simulink model "ESTteam33"  (R2024b)
settings: Solver=FixedStepAuto  StartTime=0.0  StopTime=stopt  FixedStep=deltat  MaxStep=0.05  RelTol=1e-3
InitFcn:
  | clear all;
  | close all;
  | clc;
  | 
  | % add the data and script directories
  | addpath('data','scripts');
  | 
  | % load the constants (units)
  | constants;
  | 
  | % load the simulation parameters
  | preprocessing;
StopFcn:
  | postprocessing;
values from neighbouring files (symbols this model uses):
  aExtraction = eta_extr    (= 0.8439)    [preprocessing.m]
  bStorage = 0    [preprocessing.m]
  deltat = 5*unit("min")    [preprocessing.m]
  EStorageInitial = EStorageMax/2    (= 1000000000)    [preprocessing.m]
  EStorageMax = 2*10e8    (= 2000000000)    [preprocessing.m]
  EStorageMin = EStorageMax/20    (= 100000000)    [preprocessing.m]
  eta_converter = 0.97    [preprocessing.m]
  L = 0.11 * 29    (= 3.19)    [preprocessing.m]
  L_demand = 10    [preprocessing.m]
  N_sphere = 9    [preprocessing.m]
  r_sph = 10    [preprocessing.m]
  Rprime = 0.1181    [preprocessing.m]
  V = 320e3    (= 320000)    [preprocessing.m]
settings Model: Creator=joche  LastModifiedBy=yujingze
settings DataIOCC: SaveFormat=Array  SaveOutput=off  ReturnWorkspaceOutputs=off
settings OptimizationCC: ReuseModelBlockBuffer=off
settings ModelReferenceCC: EnableRefExpFcnMdlSchedulingChecks=on
settings RTWCC: GPUComputeCapability=3.5

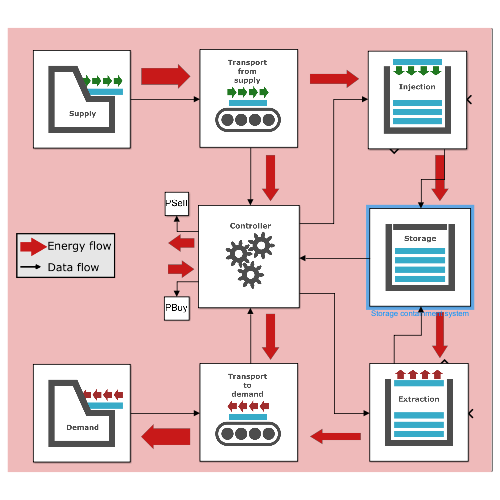
[thumbnail: Simulink's stored preview of the top-level diagram]
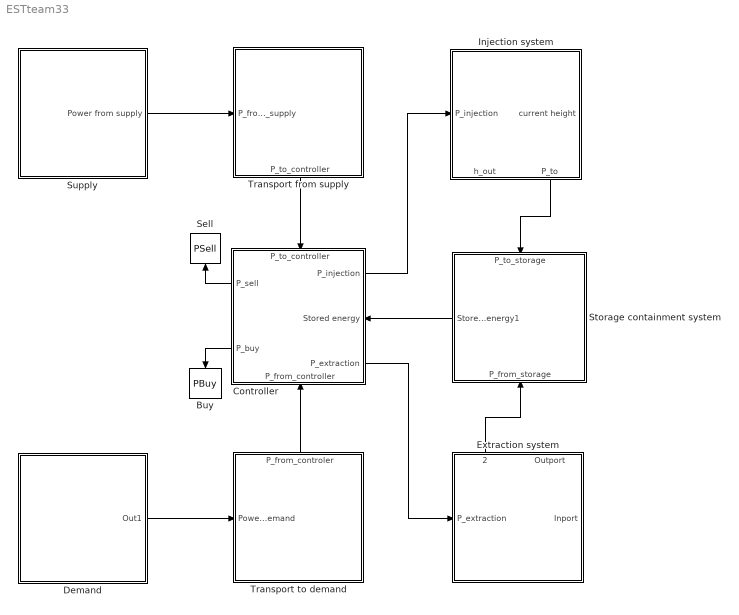
== system ESTteam33 ==
  Buy : ToWorkspace  VariableName=PBuy  SampleTime=-1
  Controller : Subsystem
      settings: PortSchema="{\"entries\":[{\"content\":{\"sides\":[{\"content\":{\"connectorIds\":[\"Out3\",\"Out4\"]},\"type\":\"ConnectorPlacement.EquallySpacedRectSide\",\"uuid\":\"4daf33ce-c96a-4783-b5c4-228eed953e01\"},{\"content\":{\"connectorIds\":[\"Out1\",\"In3\",\"Out2\"],\"side\":\"RIGHT\"},\"type\":\"ConnectorPlacement.EquallySpacedRectSide\",\"uuid\":\"e9942e50-8467-4af8-b79b-80636cbc76e5\"},{\"content\":{\"connectorIds\":[\"In1\"],\"side\":\"TOP\"},\"type\":\"ConnectorPlacement.EquallySpacedRectSide\",\"uuid\":\"f315e931-d69b-4751-b712-f89c6c81baeb\"},{\"content\":{\"connectorIds\":[\"In2\"],\"side\":\"BOTTOM\"},\"type\":\"ConnectorPlacement.EquallySpacedRectSide\",\"uuid\":\"44715ee6-5cd5-4669-bcb9-5ed7c869bdb3\"}]},\"type\":\"ConnectorPlacement.EquallySpacedConnector\",\"uuid\":\"fff48899-944b-4064-b7d7-ecc12144fb48\"}],\"packageUris\":[\"http://schema.mathworks.com/mf0/Connector/R2020b\"],\"version\":\"1.0\"}"
      mask Display: image('$imagefile'); % Use "Edit Image" on toolstrip to change.
  Demand : Subsystem
      mask Display: image('$imagefile'); % Use "Edit Image" on toolstrip to change.
  Extraction system : Subsystem
      settings: PortSchema="{\"entries\":[{\"content\":{\"sides\":[{\"content\":{\"connectorIds\":[\"In1\"]},\"type\":\"ConnectorPlacement.EquallySpacedRectSide\",\"uuid\":\"05c5933d-55fc-4e06-853f-fc26d42905f9\"},{\"content\":{\"connectorIds\":[\"In2\"],\"side\":\"RIGHT\"},\"type\":\"ConnectorPlacement.EquallySpacedRectSide\",\"uuid\":\"327426c5-31d5-498b-a2bd-83e49353408c\"},{\"content\":{\"side\":\"TOP\"},\"type\":\"ConnectorPlacement.EquallySpacedRectSide\",\"uuid\":\"55306cf3-a3de-4385-a5ae-b8600ecdd5a2\"},{\"content\":{\"connectorIds\":[\"Out1\",\"Out2\"],\"side\":\"BOTTOM\"},\"type\":\"ConnectorPlacement.EquallySpacedRectSide\",\"uuid\":\"08fcc9c3-40d3-4ac6-b914-dfeef6039ffb\"}]},\"type\":\"ConnectorPlacement.EquallySpacedConnector\",\"uuid\":\"cb35d5ba-e8c6-462c-b7b2-fe8356d4b0a1\"}],\"packageUris\":[\"http://schema.mathworks.com/mf0/Connector/R2020b\"],\"version\":\"1.0\"}"
      mask Display: image('$imagefile'); % Use "Edit Image" on toolstrip to change.
  Injection system : Subsystem
      settings: PortSchema="{\"entries\":[{\"content\":{\"sides\":[{\"content\":{\"connectorIds\":[\"In1\"]},\"type\":\"ConnectorPlacement.EquallySpacedRectSide\",\"uuid\":\"05c5933d-55fc-4e06-853f-fc26d42905f9\"},{\"content\":{\"connectorIds\":[\"In2\"],\"side\":\"RIGHT\"},\"type\":\"ConnectorPlacement.EquallySpacedRectSide\",\"uuid\":\"327426c5-31d5-498b-a2bd-83e49353408c\"},{\"content\":{\"connectorIds\":[\"Out1\",\"Out2\"],\"side\":\"TOP\"},\"type\":\"ConnectorPlacement.EquallySpacedRectSide\",\"uuid\":\"55306cf3-a3de-4385-a5ae-b8600ecdd5a2\"},{\"content\":{\"side\":\"BOTTOM\"},\"type\":\"ConnectorPlacement.EquallySpacedRectSide\",\"uuid\":\"08fcc9c3-40d3-4ac6-b914-dfeef6039ffb\"}]},\"type\":\"ConnectorPlacement.EquallySpacedConnector\",\"uuid\":\"cb35d5ba-e8c6-462c-b7b2-fe8356d4b0a1\"}],\"packageUris\":[\"http://schema.mathworks.com/mf0/Connector/R2020b\"],\"version\":\"1.0\"}"
      mask Display: image('$imagefile'); % Use "Edit Image" on toolstrip to change.
  Sell : ToWorkspace  VariableName=PSell  SampleTime=-1
  Storage containment system : Subsystem
      settings: PortSchema="{\"entries\":[{\"content\":{\"sides\":[{\"content\":{\"connectorIds\":[\"Out1\"]},\"type\":\"ConnectorPlacement.EquallySpacedRectSide\",\"uuid\":\"0ba48424-33b9-4934-970f-64fe5d8b070e\"},{\"content\":{\"side\":\"RIGHT\"},\"type\":\"ConnectorPlacement.EquallySpacedRectSide\",\"uuid\":\"9cde340f-8f39-4499-9a12-5e1623737660\"},{\"content\":{\"connectorIds\":[\"In1\"],\"side\":\"TOP\"},\"type\":\"ConnectorPlacement.EquallySpacedRectSide\",\"uuid\":\"2af8db04-7fd0-4902-8637-8dc00edb4598\"},{\"content\":{\"connectorIds\":[\"In2\"],\"side\":\"BOTTOM\"},\"type\":\"ConnectorPlacement.EquallySpacedRectSide\",\"uuid\":\"e21ea806-d777-41a3-a53f-556fae66854b\"}]},\"type\":\"ConnectorPlacement.EquallySpacedConnector\",\"uuid\":\"4e2ddb36-4db3-4ab4-858b-ebb8ccefeb1f\"}],\"packageUris\":[\"http://schema.mathworks.com/mf0/Connector/R2020b\"],\"version\":\"1.0\"}"
      mask Display: image('$imagefile'); % Use "Edit Image" on toolstrip to change.
  Supply : Subsystem
      mask Display: image('$imagefile'); % Use "Edit Image" on toolstrip to change.
  Transport from supply : Subsystem
      settings: PortSchema="{\"entries\":[{\"content\":{\"sides\":[{\"content\":{\"connectorIds\":[\"In1\"]},\"type\":\"ConnectorPlacement.EquallySpacedRectSide\",\"uuid\":\"31329006-3d36-4d93-9c44-7503a515d397\"},{\"content\":{\"connectorIds\":[],\"side\":\"RIGHT\"},\"type\":\"ConnectorPlacement.EquallySpacedRectSide\",\"uuid\":\"aba139c7-f9b6-4881-a56b-a4cbbedacd88\"},{\"content\":{\"connectorIds\":[],\"side\":\"TOP\"},\"type\":\"ConnectorPlacement.EquallySpacedRectSide\",\"uuid\":\"e683eb73-7a35-4160-9c39-da83856a6278\"},{\"content\":{\"connectorIds\":[\"Out1\"],\"side\":\"BOTTOM\"},\"type\":\"ConnectorPlacement.EquallySpacedRectSide\",\"uuid\":\"1170dd18-447c-437f-9043-6812c2877331\"}]},\"type\":\"ConnectorPlacement.EquallySpacedConnector\",\"uuid\":\"804af608-1d70-444f-af69-e05f19bf98f3\"}],\"packageUris\":[\"http://schema.mathworks.com/mf0/Connector/R2020b\"],\"version\":\"1.0\"}"
      mask Display: image('$imagefile'); % Use "Edit Image" on toolstrip to change.
  Transport to demand : Subsystem
      settings: PortSchema="{\"entries\":[{\"content\":{\"sides\":[{\"content\":{\"connectorIds\":[\"In1\"]},\"type\":\"ConnectorPlacement.EquallySpacedRectSide\",\"uuid\":\"31329006-3d36-4d93-9c44-7503a515d397\"},{\"content\":{\"connectorIds\":[],\"side\":\"RIGHT\"},\"type\":\"ConnectorPlacement.EquallySpacedRectSide\",\"uuid\":\"aba139c7-f9b6-4881-a56b-a4cbbedacd88\"},{\"content\":{\"connectorIds\":[\"Out1\"],\"side\":\"TOP\"},\"type\":\"ConnectorPlacement.EquallySpacedRectSide\",\"uuid\":\"e683eb73-7a35-4160-9c39-da83856a6278\"},{\"content\":{\"connectorIds\":[],\"side\":\"BOTTOM\"},\"type\":\"ConnectorPlacement.EquallySpacedRectSide\",\"uuid\":\"c378138f-7233-4483-870c-40a69b3495ee\"}]},\"type\":\"ConnectorPlacement.EquallySpacedConnector\",\"uuid\":\"804af608-1d70-444f-af69-e05f19bf98f3\"}],\"packageUris\":[\"http://schema.mathworks.com/mf0/Connector/R2020b\"],\"version\":\"1.0\"}"
      mask Display: image('$imagefile'); % Use "Edit Image" on toolstrip to change.
  wires:
  Supply/1(Power from supply) -> Transport from supply/1(P_from_supply)
  Transport from supply/1(P_to_controller) -> Controller/1(P_to_controller)
  Transport to demand/1(P_from_controler) -> Controller/2(P_from_controller)
  Demand/1(Out1) -> Transport to demand/1(Power to demand)
  Controller/3(P_sell) -> Sell/1
  Controller/2(P_extraction) -> Extraction system/2(P_extraction)
  Injection system/1(P_to) -> Storage containment system/1(P_to_storage)
  Extraction system/2(P_from_storage) -> Storage containment system/2(P_from_storage)
  Storage containment system/1(Stored energy1) -> Controller/3(Stored energy)
  Controller/1(P_injection) -> Injection system/2(P_injection)
  Controller/4(P_buy) -> Buy/1

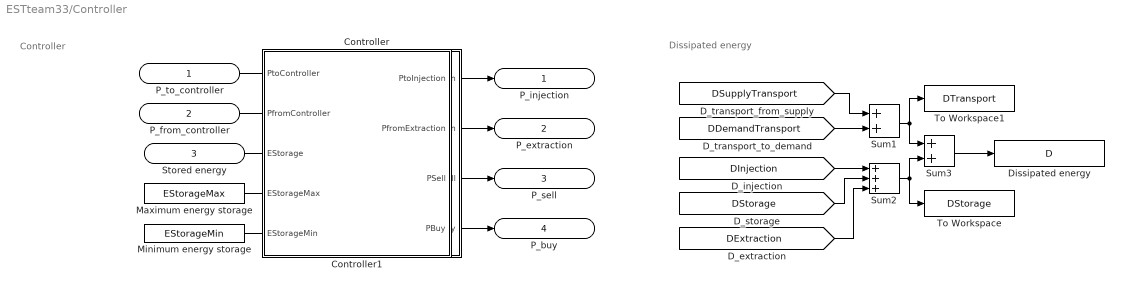
== system ESTteam33/Controller ==
  note: Dissipated energy
  note: Controller
  P_to_controller : Inport
  P_from_controller : Inport  Port=2
  Stored energy : Inport  Port=3
  Controller : MATLAB Function  TreatAsAtomicUnit=on
  Controller1 : MATLAB Function  TreatAsAtomicUnit=on
  Dissipated energy : ToWorkspace  VariableName=D  SampleTime=-1
  Maximum energy storage : Constant  Value=EStorageMax
  Minimum energy storage : Constant  Value=EStorageMin
  Sum1 : Sum
  Sum2 : Sum  Inputs=+++
  Sum3 : Sum
  To Workspace : ToWorkspace  VariableName=DStorage  SampleTime=-1
  To Workspace1 : ToWorkspace  VariableName=DTransport  SampleTime=-1
  P_injection : Outport
  P_extraction : Outport  Port=2
  P_sell : Outport  Port=3
  P_buy : Outport  Port=4
  wires:
  P_from_controller/1 -> Controller/2(PfromController)
  Controller/2(PfromExtraction) -> P_extraction/1
  Controller/3(PSell) -> P_sell/1
  Controller/4(PBuy) -> P_buy/1
  Minimum energy storage/1 -> Controller/5(EStorageMin)
  Maximum energy storage/1 -> Controller/4(EStorageMax)
  P_to_controller/1 -> Controller/1(PtoController)
  Controller/1(PtoInjection) -> P_injection/1
  Stored energy/1 -> Controller/3(EStorage)
  [DDemandTransport] -> Sum1/2
  [DSupplyTransport] -> Sum1/1
  [DInjection] -> Sum2/1
  [DStorage] -> Sum2/2
  [DExtraction] -> Sum2/3
  Sum2/1 -> To Workspace/1, Sum3/2
  Sum1/1 -> To Workspace1/1, Sum3/1
  Sum3/1 -> Dissipated energy/1

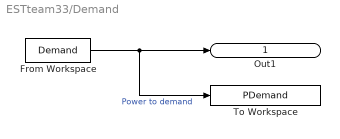
== system ESTteam33/Demand ==
  From Workspace : FromWorkspace  VariableName=Demand  OutputAfterFinalValue=Setting to zero
  To Workspace : ToWorkspace  VariableName=PDemand  SampleTime=-1
  Out1 : Outport
  wires:
  From Workspace/1 -> To Workspace/1, Out1/1  "Power to demand"

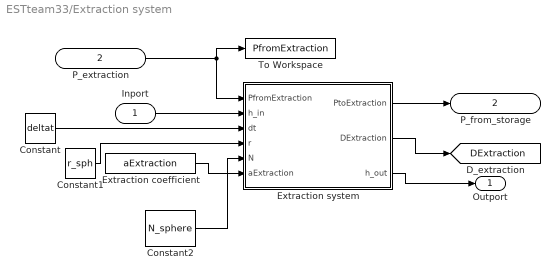
== system ESTteam33/Extraction system ==
  Inport : Inport
  P_extraction : Inport  Port=2
  Constant : Constant  Value=deltat
  Constant1 : Constant  Value=r_sph
  Constant2 : Constant  Value=N_sphere
  Extraction coefficient : Constant  Value=aExtraction
  Extraction system : MATLAB Function  TreatAsAtomicUnit=on
  To Workspace : ToWorkspace  VariableName=PfromExtraction  SampleTime=-1
  Outport : Outport
  P_from_storage : Outport  Port=2
  tag scope: DExtraction=global
  wires:
  P_extraction/1 -> Extraction system/1(PfromExtraction), To Workspace/1
  Extraction system/1(PtoExtraction) -> P_from_storage/1
  Extraction coefficient/1 -> Extraction system/6(aExtraction)
  Extraction system/2(DExtraction) -> [DExtraction]
  Inport/1 -> Extraction system/2(h_in)
  Extraction system/3(h_out) -> Outport/1
  Constant/1 -> Extraction system/3(dt)
  Constant2/1 -> Extraction system/5(N)
  Constant1/1 -> Extraction system/4(r)

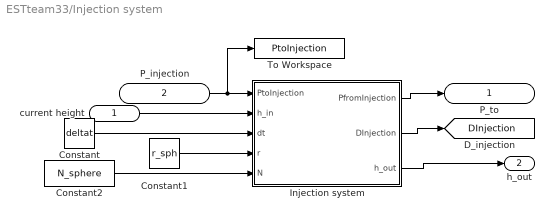
== system ESTteam33/Injection system ==
  current height : Inport
  P_injection : Inport  Port=2
  Constant : Constant  Value=deltat
  Constant1 : Constant  Value=r_sph
  Constant2 : Constant  Value=N_sphere
  Injection system : MATLAB Function  TreatAsAtomicUnit=on
  To Workspace : ToWorkspace  VariableName=PtoInjection  SampleTime=-1
  P_to : Outport
  h_out : Outport  Port=2
  tag scope: DInjection=global
  wires:
  P_injection/1 -> To Workspace/1, Injection system/1(PtoInjection)
  Injection system/1(PfromInjection) -> P_to/1
  Injection system/2(DInjection) -> [DInjection]
  Injection system/3(h_out) -> h_out/1
  current height/1 -> Injection system/2(h_in)
  Constant/1 -> Injection system/3(dt)
  Constant2/1 -> Injection system/5(N)
  Constant1/1 -> Injection system/4(r)

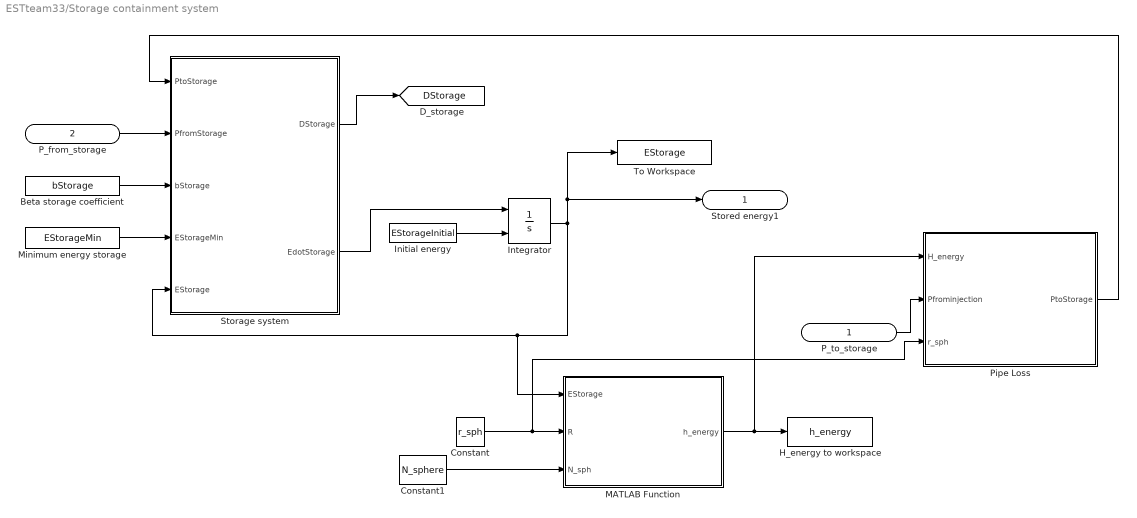
== system ESTteam33/Storage containment system ==
  P_to_storage : Inport
  P_from_storage : Inport  Port=2
  Beta storage coefficient : Constant  Value=bStorage
  Constant : Constant  Value=r_sph
  Constant1 : Constant  Value=N_sphere
  H_energy to workspace : ToWorkspace  VariableName=h_energy  SaveFormat=Timeseries  SampleTime=-1
  Initial energy : Constant  Value=EStorageInitial
  Integrator : Integrator  InitialConditionSource=external  LimitOutput=on  UpperSaturationLimit=EStorageMax  LowerSaturationLimit=0
  MATLAB Function : MATLAB Function  TreatAsAtomicUnit=on
  Minimum energy storage : Constant  Value=EStorageMin
  Pipe Loss : MATLAB Function  TreatAsAtomicUnit=on
  Storage system : MATLAB Function  TreatAsAtomicUnit=on
  To Workspace : ToWorkspace  VariableName=EStorage  SampleTime=-1
  Stored energy1 : Outport
  tag scope: DStorage=global
  wires:
  P_from_storage/1 -> Storage system/2(PfromStorage)
  Storage system/1(DStorage) -> [DStorage]
  Beta storage coefficient/1 -> Storage system/3(bStorage)
  Storage system/2(EdotStorage) -> Integrator/1
  Minimum energy storage/1 -> Storage system/4(EStorageMin)
  Initial energy/1 -> Integrator/2
  Integrator/1 -> To Workspace/1, Stored energy1/1, MATLAB Function/1(EStorage), Storage system/5(EStorage)
  Constant1/1 -> MATLAB Function/3(N_sph)
  Constant/1 -> Pipe Loss/3(r_sph), MATLAB Function/2(R)
  MATLAB Function/1(h_energy) -> Pipe Loss/1(H_energy), H_energy to workspace/1
  P_to_storage/1 -> Pipe Loss/2(Pfrominjection)
  Pipe Loss/1(PtoStorage) -> Storage system/1(PtoStorage)

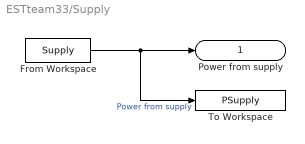
== system ESTteam33/Supply ==
  From Workspace : FromWorkspace  VariableName=Supply  OutputAfterFinalValue=Setting to zero
  To Workspace : ToWorkspace  VariableName=PSupply  SampleTime=-1
  Power from supply : Outport
  wires:
  From Workspace/1 -> To Workspace/1, Power from supply/1  "Power from supply"

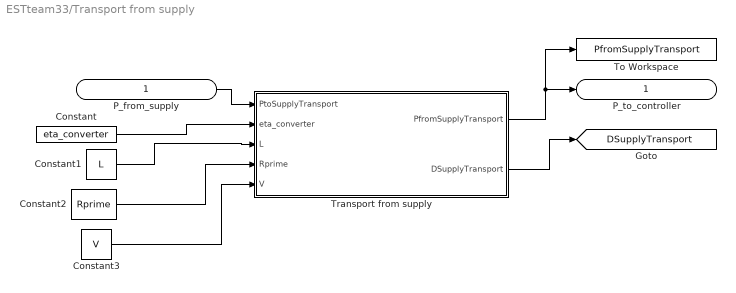
== system ESTteam33/Transport from supply ==
  P_from_supply : Inport
  Constant : Constant  Value=eta_converter
  Constant1 : Constant  Value=L
  Constant2 : Constant  Value=Rprime
  Constant3 : Constant  Value=V
  To Workspace : ToWorkspace  VariableName=PfromSupplyTransport  SampleTime=-1
  Transport from supply : MATLAB Function  TreatAsAtomicUnit=on
  P_to_controller : Outport
  tag scope: DSupplyTransport=global
  wires:
  P_from_supply/1 -> Transport from supply/1(PtoSupplyTransport)
  Transport from supply/1(PfromSupplyTransport) -> To Workspace/1, P_to_controller/1
  Transport from supply/2(DSupplyTransport) -> [DSupplyTransport]
  Constant/1 -> Transport from supply/2(eta_converter)
  Constant1/1 -> Transport from supply/3(L)
  Constant2/1 -> Transport from supply/4(Rprime)
  Constant3/1 -> Transport from supply/5(V)

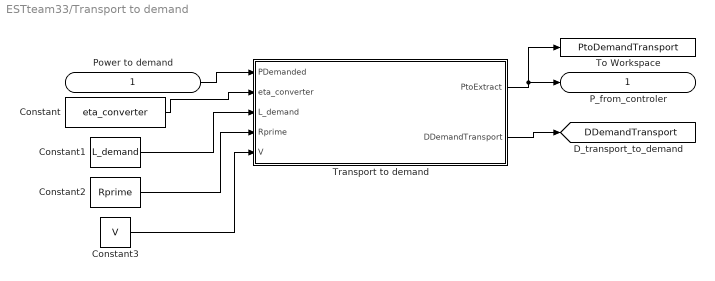
== system ESTteam33/Transport to demand ==
  Power to demand : Inport
  Constant : Constant  Value=eta_converter
  Constant1 : Constant  Value=L_demand
  Constant2 : Constant  Value=Rprime
  Constant3 : Constant  Value=V
  To Workspace : ToWorkspace  VariableName=PtoDemandTransport  SampleTime=-1
  Transport to demand : MATLAB Function  TreatAsAtomicUnit=on
  P_from_controler : Outport
  tag scope: DDemandTransport=global
  wires:
  Power to demand/1 -> Transport to demand/1(PDemanded)
  Transport to demand/1(PtoExtract) -> To Workspace/1, P_from_controler/1
  Transport to demand/2(DDemandTransport) -> [DDemandTransport]
  Constant/1 -> Transport to demand/2(eta_converter)
  Constant1/1 -> Transport to demand/3(L_demand)
  Constant2/1 -> Transport to demand/4(Rprime)
  Constant3/1 -> Transport to demand/5(V)

== matlab function ESTteam33/Transport to demand/Transport to demand ==
  data: PDemanded input; PtoExtract output; eta_converter input; DDemandTransport output; L_demand input; Rprime input; V input
function [PtoExtract, DDemandTransport] = demandTransport(PDemanded, eta_converter, L_demand, Rprime, V)
% Inputs:
% P_Demanded : Power you want to reach the grid (W)
% eta         : Efficiency of conversion stages (0 < eta <= 1)
% L_transp_demand: Cable length (km)
% R_prime     : Resistance per unit length (Ohm/km)
% V           : Voltage (Volts)

% Output:
% PtoExtract  : Power needed before losses (W)

% Coefficients for the quadratic equation:
% a*P_required^2 + b*P_required + c = 0

a = (eta_converter^3) * L_demand * Rprime / V^2;
b = -eta_converter^2;
c = PDemanded;

% Discriminant
D = b^2 - 4*a*c;

% Check for non-negative discriminant to avoid complex results
    if D < 0
    PtoExtract = 0; % or raise an error/warning depending on application
        else
        % Only the positive root makes physical sense
            P1 = (-b + sqrt(D)) / (2*a);
            P2 = (-b - sqrt(D)) / (2*a);
        

       if P1 > 0 && P2 > 0
    if P1 > P2
        PtoExtract = P2;
    else
        PtoExtract = P1;
    end
elseif P1 > 0
    PtoExtract = P1;
elseif P2 > 0
    PtoExtract = P2;
else
    PtoExtract = 0; % Both roots are non-positive
end
    end
DDemandTransport = PtoExtract - PDemanded;
end

== matlab function ESTteam33/Storage containment system/MATLAB Function ==
  data: EStorage input; h_energy output; R input; N_sph input
function h_energy = computeHeightFromEnergy(EStorage, R, N_sph)
% computeStartHeightFromEnergy : Solves for initial water height in spherical tanks
% given total stored energy.
%
% Inputs:
%   EStorage  : Total energy stored [J]
%   R         : Radius of spherical tank [m]
%   N_sph     : Number of spherical tanks
%   Hturbine  : Turbine elevation reference [m]
%   rho       : Water density [kg/m^3]
%   g         : Gravitational acceleration [m/s^2]
%
% Output:
%   h         : Water height in tank corresponding to E_start [m]
rho = 1000;        % Water density [kg/m^3]
g = 9.81;          % Gravitational acceleration [m/s^2]
depth = 100;


    Hturbine = depth - R; %Gives the average head
    % Anonymous function: Computes total energy for a given height
    energyFromHeight = @(h_energy) N_sph * rho * g * ...
        ((pi * h_energy.^2 .* (3*R - h_energy)) / 3) .* (Hturbine + (R - (h_energy / 3) .* (3 - h_energy / R)));

    % Objective: Find height such that energyFromHeight(h) = E_start
    % Use fzero or fminsearch if fsolve is not available
    h_guess = R; % initial guess (half full)
    options = optimset('Display','off');
    
    % Define function to zero
    f = @(h_energy) energyFromHeight(h_energy) - EStorage;

    % Use fzero to find root in a valid range
    h_energy = fzero(f, [0, 2*R], options);
end

== matlab function ESTteam33/Storage containment system/Pipe Loss ==
  data: PtoStorage output; H_energy input; Pfrominjection input; r_sph input
function PtoStorage = PipeLossFunction(H_energy, Pfrominjection,r_sph)
    % Physical parameters
    rho = 1000;         % [kg/m^3]
    g = 9.8;            % [m/s^2]
    mu = 1.1e-3;        % [Pa·s]
    epsilon = 0.015e-3; % [m]

    % Pipe geometry
    L = 4.5+4*r_sph;           % [m]
    D = 1.0;            % [m]
    A = pi * (D / 2)^2; % [m^2]
    
    % Minor loss coefficients
    K_total = 0.3 + 0.15 + 0.5 + 1.0; % elbows + valve + entry + exit

    % Head available from pressure
    H_avail = 100 - H_energy;
if Pfrominjection~=0
    % Get Volumetric flow from P
    Q=Pfrominjection/(rho*g*H_avail)
    V=Q/A
    Re = rho * V * D / mu ;

 % Friction factor
    if Re < 2300
    f = 64 / Re ; % Laminar flow
    else
    f = 0.25 / ( log10 ( epsilon /(3.7* D ) + 5.74/ Re ^0.9) ) ^2;
    end        
    h_major = f * (L / D) * (V^2) / (2 * g);
    h_minor = K_total * (V^2) / (2 * g);
    H_losses = h_major + h_minor;
    H_net = H_avail - H_losses;

    % Final power to storage (zero if H_net = 0)
    PtoStorage = rho * g * Q * H_net;
else
    PtoStorage=0
end
end

== matlab function ESTteam33/Injection system/Injection system ==
  data: PtoInjection input; h_in input; PfromInjection output; dt input; DInjection output; h_out output; r input; N input

function [PfromInjection, DInjection, h_out] = computeInjectionSimulink(PtoInjection, h_in, dt,r,N)
% Calculates stored power, loss, and new tank height from pump input

 % Physical constants
    rho = 1000;          % Water density [kg/m^3]
    g = 9.81;            % Gravity [m/s^2]
    r_sph_small  = r;
    N_small = N;
    depth = 100;
% Pump and converter efficiency
eta_converter = 0.97;
eta_pump = 0.80;
eta_inj = eta_converter * eta_pump;

H_eff = depth - h_in;

% Pumped mass (kg): m = (eta * P * dt) / (g * H_eff)
m_pumped = eta_inj * PtoInjection * dt / (g * H_eff);
V_pumped = m_pumped / rho;   % [m^3]

% Total tank cross-sectional volume at this height
% For inverse spherical cap: use differential volume approximation
% Instead, solve new height numerically (simplified here)

% Add volume to tank (assuming uniform distribution)
V_total = (pi * h_in^2 * (3*r_sph_small - h_in)) / 3 + V_pumped / N_small;


% Solve for new height from volume
% Use Newton-Raphson or brute-force (we’ll use simple loop approx here)
h_out = h_in;
for i = 1:10
    V_guess = (pi * h_out^2 * (3*r_sph_small - h_out)) / 3;
    error = V_guess - V_total;
    dVdh = pi * h_out * (3*r_sph_small - h_out); % derivative dV/dh
    h_out = h_out - error / dVdh;
    h_out = max(0, min(h_out, 2 * r_sph_small));
end

% Potential energy added
E_added = m_pumped * g * H_eff;
PfromInjection = E_added / dt;
DInjection = PtoInjection - PfromInjection;
end

== matlab function ESTteam33/Transport from supply/Transport from supply ==
  data: PtoSupplyTransport input; PfromSupplyTransport output; eta_converter input; DSupplyTransport output; L input; Rprime input; V input
function [PfromSupplyTransport, DSupplyTransport] = supplyTransport(PtoSupplyTransport, eta_converter, L, Rprime, V)
    % supplyTransport: Calculates power delivered after transport, considering losses
    % PtoSupplyTransport : Power intended to be transported [W]
    % eta                : Transformer efficiency
    % L                  : Cable length [km]
    % Rprime             : Resistance per unit length [Ohm/km]
    % V                  : Transmission voltage [V]
    % Returns:
    % PfromSupplyTransport : Power delivered after transport [W]
    % DSupplyTransport     : Total power losses during transport [W]

    % Calculate power after transport using the formula
    PfromSupplyTransport = eta_converter^2 * PtoSupplyTransport - eta_converter^3 * L * Rprime * (PtoSupplyTransport^2) / (V^2);

    % Calculate the total losses
    DSupplyTransport = PtoSupplyTransport - PfromSupplyTransport;
end

== matlab function ESTteam33/Controller/Controller ==
  data: PtoInjection output; PfromExtraction output; PSell output; PBuy output; PtoController input; PfromController input; EStorage input; EStorageMax input; EStorageMin input
function [PtoInjection, PfromExtraction, PSell, PBuy] = controller(PtoController, PfromController, EStorage, EStorageMax, EStorageMin)
    
    %% Power surplus or deficit

    deltaP = PtoController - PfromController;

    % Power surplus
    if deltaP >= 0

        %% Storage injection

        % Storage system is not full
        if EStorage < EStorageMax 

            PtoInjection = deltaP;

        % Storage system is full
        else
            PtoInjection = 0;
        end

        %% Storage extraction

        PfromExtraction = 0;

        %% Load-balancing
        PSell   = deltaP - PtoInjection;
        PBuy    = 0;

    % Power deficit
    else

        %% Storage injection

        PtoInjection = 0;

        %% Storage extraction

        % Storage system is not empty
        if EStorage > EStorageMin

            PfromExtraction = -deltaP;

        % Storage system is empty
        else
            PfromExtraction = 0;
        end

        %% Load-balancing

        PSell = 0;
        PBuy  = -deltaP - PfromExtraction;
    end

== matlab function ESTteam33/Extraction system/Extraction system ==
  data: PfromExtraction input; h_in input; dt input; r input; N input; PtoExtraction output; aExtraction input; DExtraction output; h_out output
function [PtoExtraction, DExtraction, h_out] = extraction(PfromExtraction, h_in, dt, r, N, aExtraction)
% Computes electrical power output and updated tank height from water inflow (turbine extraction)

    % Physical constants
    rho = 1000;      % Water density [kg/m^3]
    g = 9.81;        % Gravitational acceleration [m/s^2]
    depth = 100;     % Height of upper reservoir relative to seabed [m]

    % Tank geometry
    r_sph = r;
    N_sphere = N;

    % Turbine efficiency
    eta_extr = aExtraction;

    % Effective head: height difference 
    h = h_in;
    H_eff = depth - h;

    % Hydraulic energy input
    E_hydraulic = PfromExtraction * dt;

    % Mass of water needed to extract this energy
    m_water = E_hydraulic / (g * H_eff);
    V_water = m_water / rho;
    V_water_per_tank = V_water / N_sphere;

    % Initial volume
    V_initial = (pi * h^2 * (3 * r_sph - h)) / 3;
    V_total = V_initial + V_water_per_tank;

    % Solve for new height using Newton-Raphson
    h_out = h;
    for i = 1:10
        V_guess = (pi * h_out^2 * (3 * r_sph - h_out)) / 3;
        error = V_guess - V_total;
        dVdh = pi * h_out * (3 * r_sph - h_out);
        h_out = h_out - error / dVdh;
        h_out = max(0, min(h_out, 2 * r_sph));
    end

    % Electrical output
    E_electric = E_hydraulic * eta_extr;
    PtoExtraction = E_electric / dt;

    % Losses
    DExtraction = PfromExtraction - PtoExtraction;
end

== matlab function ESTteam33/Storage containment system/Storage system ==
  settings: updateMethod=DISCRETE
  data: DStorage output; EdotStorage output; PtoStorage input; PfromStorage input; bStorage input; EStorageMin input; EStorage input
function [DStorage, EdotStorage] = Storage(PtoStorage, PfromStorage, bStorage, EStorageMin, EStorage)
% Storage : Models storage self-discharge and energy rate of change
% PtoStorage   : Power input to storage [W]
% PfromStorage : Power output from storage [W]
% bStorage     : Storage dissipation coefficient [1/s]
% EStorageMin  : Minimum storage energy [J]
% EStorage     : Current storage energy [J]
% h_inin, h_inex : Heights from injection and extraction

% Storage power loss and energy change
DStorage = bStorage * (EStorage - EStorageMin);
EdotStorage = PtoStorage - PfromStorage - DStorage;
end

== matlab function ESTteam33/Controller/Controller1 ==
  data: PtoInjection output; PfromExtraction output; PSell output; PBuy output; PtoController input; PfromController input; EStorage input; EStorageMax input; EStorageMin input
function [PtoInjection, PfromExtraction, PSell, PBuy] = controller(PtoController, PfromController, EStorage, EStorageMax, EStorageMin)
    
    %% Power surplus or deficit
    dt = 900;
    deltaP = PtoController - PfromController;
   
    % Power surplus
    if deltaP >= 0

        %% Storage injection
        
        % Storage system is not full 
        if (EStorageMax - EStorage) > 0
            if (deltaP > (EStorageMax - EStorage))
                PtoInjection = (EStorageMax - EStorage) / dt;
            else
                PtoInjection = deltaP;
            end
        else
            PtoInjection = 0;
        end

        %% Storage extraction

        PfromExtraction = 0;

        %% Load-balancing
        PSell   = deltaP - PtoInjection;
        PBuy    = 0;

    % Power deficit
    else

        %% Storage injection

        PtoInjection = 0;

        %% Storage extraction

        % Storage system is not empty and can supply deltaP
        if (EStorage - deltaP) > EStorageMin
            PfromExtraction = -deltaP;
        elseif (EStorage - EStorageMin) > 0 % not empty but not enough to meet all demand
            PfromExtraction = (EStorage - EStorageMin) / dt;
        else
            PfromExtraction = 0; % empty
        end

        %% Load-balancing

        PSell = 0;
        PBuy  = -deltaP - PfromExtraction;
    end
